simulink model "c_simulink_start"  (R2016b)
settings: Solver=FixedStepAuto  StartTime=0.0  StopTime=40  FixedStep=0.01  RelTol=1e-3
settings Model: Creator=USER  LastModifiedBy=USER
settings OptimizationCC: DefaultParameterBehavior=Inlined
settings DebuggingCC: ParameterTunabilityLossMsg=error
settings SFSimCC: SimCustomInitializer=Filter_Init();  SimUserSources=filter.c
settings SFSimCC: SimCustomHeaderCode=|
  | extern void Filter_Init(void);
  | extern double Filter_UpdateY(double x);
settings RTWCC: GenerateReport=on  CustomInitializer=Filter_Init();  LaunchReport=on
settings CodeAppCC: ForceParamTrailComments=on  OperatorAnnotations=on  MATLABSourceComments=on

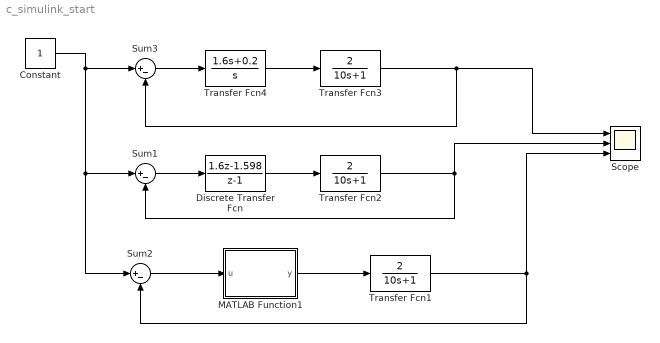
== system c_simulink_start ==
  Constant : Constant
  Discrete Transfer Fcn : DiscreteTransferFcn  Numerator=[1.6 -1.598]  Denominator=[1 -1]  SampleTime=0.01
  MATLAB Function1 : MATLAB Function  TreatAsAtomicUnit=on  SystemSampleTime=0.01
  Scope : Scope  NumInputPorts=3
  Sum1 : Sum  Inputs=|+-
  Sum2 : Sum  Inputs=|+-
  Sum3 : Sum  Inputs=|+-
  Transfer Fcn1 : TransferFcn  Numerator=[2]  Denominator=[10 1]
  Transfer Fcn2 : TransferFcn  Numerator=[2]  Denominator=[10 1]
  Transfer Fcn3 : TransferFcn  Numerator=[2]  Denominator=[10 1]
  Transfer Fcn4 : TransferFcn  Numerator=[1.6 0.2]  Denominator=[1 0]
  wires:
  Constant/1 -> Sum3/1, Sum2/1, Sum1/1
  Sum1/1 -> Discrete Transfer Fcn/1
  Transfer Fcn2/1 -> Scope/2, Sum1/2
  Transfer Fcn1/1 -> Sum2/2, Scope/3
  Discrete Transfer Fcn/1 -> Transfer Fcn2/1
  MATLAB Function1/1(y) -> Transfer Fcn1/1
  Sum2/1 -> MATLAB Function1/1(u)
  Transfer Fcn4/1 -> Transfer Fcn3/1
  Transfer Fcn3/1 -> Sum3/2, Scope/1
  Sum3/1 -> Transfer Fcn4/1

== matlab function c_simulink_start/MATLAB Function1 ==
  data: u input; y output
function y = fcn(u)
y=double(0);
y = coder.ceval('Filter_UpdateY',u);
